simulink model "SecRwLtStBkReclnIsPosChk"  (R2024b)
settings: Solver=FixedStepDiscrete  StartTime=0.0  StopTime=10.0  FixedStep=0.01  RelTol=1e-3
undefined symbols (not defined in the file or in its folder): KeSMSuSecRwStBackPosDelta_Val, KeSMSuSecRwStBackPosTolr_Val, KeSMSuVehicleModelConfig_Val
libraries: StIsPosChkLib x13, simulink x7
(part 2 of 2)

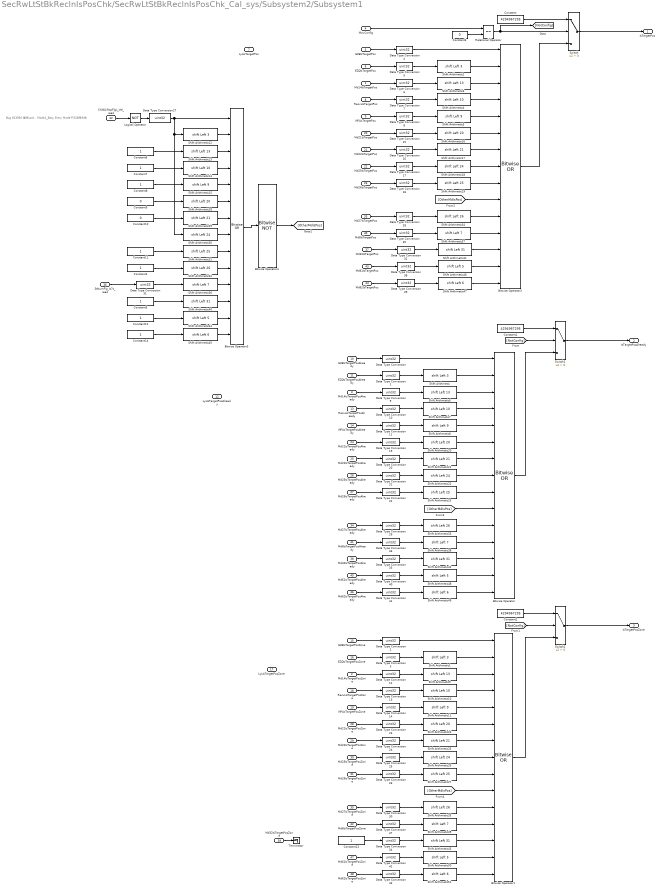
== system SecRwLtStBkReclnIsPosChk/SecRwLtStBkReclnIsPosChk_Cal_sys/Subsystem2/Subsystem1 ==
  note: Bug 813950 童锁Lock，Mode1_Easy Entry Mode 不应调用失败
  Md14IsTargetPos : Inport
  Md14IsTargetPosZone : Inport  Port=2
  Md14IsTargetPosAlready : Inport  Port=3
  MovConfig : Inport  Port=4
  EZEIsTargetPos : Inport  Port=5
  EZQIsTargetPos : Inport  Port=6
  LyLIsTargetPos : Inport  Port=7
  RecvLIsTargetPos : Inport  Port=8
  VIPLIsTargetPos : Inport  Port=9
  EZEIsTargetPosAlready : Inport  Port=10
  EZQIsTargetPosAlready : Inport  Port=11
  LyLIsTargetPosAlready : Inport  Port=12
  RecvLIsTargetPosAlready : Inport  Port=13
  VIPLIsTargetPosAlready : Inport  Port=14
  EZEIsTargetPosZone : Inport  Port=15
  EZQIsTargetPosZone : Inport  Port=16
  LyLIsTargetPosZone : Inport  Port=17
  RecvLIsTargetPosZone : Inport  Port=18
  VIPLIsTargetPosZone : Inport  Port=19
  Md21IsTargetPos : Inport  Port=20
  Md22IsTargetPos : Inport  Port=21
  Md25IsTargetPos : Inport  Port=22
  Md26IsTargetPos : Inport  Port=23
  Md21IsTargetPosAlready : Inport  Port=24
  Md22IsTargetPosAlready : Inport  Port=25
  Md25IsTargetPosAlready : Inport  Port=26
  Md26IsTargetPosAlready : Inport  Port=27
  Md21IsTargetPosZone : Inport  Port=28
  Md22IsTargetPosZone : Inport  Port=29
  Md25IsTargetPosZone : Inport  Port=30
  Md26IsTargetPosZone : Inport  Port=31
  ChldLkRspFlgL_Val_read : Inport  Port=32
  Md27IsTargetPos : Inport  Port=33
  Md27IsTargetPosAlready : Inport  Port=34
  Md27IsTargetPosZone : Inport  Port=35
  StNumFlg_Is7s_read : Inport  Port=36
  Md32IsTargetPos : Inport  Port=37
  Md32IsTargetPosAlready : Inport  Port=38
  Md32IsTargetPosZone : Inport  Port=39
  Md8IsTargetPos : Inport  Port=40
  Md8IsTargetPosAlready : Inport  Port=41
  Md8IsTargetPosZone : Inport  Port=42
  Md61IsTargetPos : Inport  Port=43
  Md62IsTargetPos : Inport  Port=44
  Md61IsTargetPosAlready : Inport  Port=45
  Md62IsTargetPosAlready : Inport  Port=46
  Md61IsTargetPosZone : Inport  Port=47
  Md62IsTargetPosZone : Inport  Port=48
  Bitwise Operator : simulink/Logic and Bit Operations/Bitwise Operator  logicop=OR  UseBitMask=off  NumInputPorts=15  BitMask=bin2dec('11011001')  BitMaskRealWorld=Stored Integer
  Bitwise Operator1 : simulink/Logic and Bit Operations/Bitwise Operator  logicop=OR  UseBitMask=off  NumInputPorts=15  BitMask=bin2dec('11011001')  BitMaskRealWorld=Stored Integer
  Bitwise Operator2 : simulink/Logic and Bit Operations/Bitwise Operator  logicop=OR  UseBitMask=off  NumInputPorts=15  BitMask=bin2dec('11011001')  BitMaskRealWorld=Stored Integer
  Bitwise Operator3 : simulink/Logic and Bit Operations/Bitwise Operator  logicop=OR  UseBitMask=off  NumInputPorts=14  BitMask=bin2dec('11011001')  BitMaskRealWorld=Stored Integer
  Bitwise Operator4 : simulink/Logic and Bit Operations/Bitwise Operator  logicop=NOT  UseBitMask=off  BitMask=bin2dec('11011001')  BitMaskRealWorld=Stored Integer
  Constant : Constant  Value=4294967295  OutDataTypeStr=uint32
  Constant1 : Constant  Value=4294967295  OutDataTypeStr=uint32
  Constant10 : Constant  Value=0  OutDataTypeStr=uint32
  Constant{4..8,11..14} (9 alike) : Constant  OutDataTypeStr=uint32
  Constant2 : Constant  Value=4294967295  OutDataTypeStr=uint32
  Constant3 : Constant  Value=0  OutDataTypeStr=uint8
  Constant9 : Constant  Value=0  OutDataTypeStr=uint32
  Data Type Conversion{,1..43} (44 alike) : DataTypeConversion  OutDataTypeStr=uint32  SaturateOnIntegerOverflow=off  RndMeth=Floor
  Logical Operator : Logic  Operator=NOT  AllPortsSameDT=off  OutDataTypeStr=boolean
  Relational Operator : RelationalOperator  Operator===  OutDataTypeStr=boolean  RndMeth=Simplest  InputSameDT=off
  Shift Arithmetic{,1..2,12} (4 alike) : ArithShift  BitShiftNumber=3  BitShiftDirection=Left
  Shift Arithmetic{4,7,10,14} (4 alike) : ArithShift  BitShiftNumber=10  BitShiftDirection=Left
  Shift Arithmetic{5,8,11,15} (4 alike) : ArithShift  BitShiftNumber=9  BitShiftDirection=Left
  Shift Arithmetic{3,6,9,13} (4 alike) : ArithShift  BitShiftNumber=13  BitShiftDirection=Left
  Shift Arithmetic{16,20,24,28} (4 alike) : ArithShift  BitShiftNumber=20  BitShiftDirection=Left
  Shift Arithmetic{17,21,25,29} (4 alike) : ArithShift  BitShiftNumber=21  BitShiftDirection=Left
  Shift Arithmetic{18,22,26,30} (4 alike) : ArithShift  BitShiftNumber=24  BitShiftDirection=Left
  Shift Arithmetic{19,23,27,31} (4 alike) : ArithShift  BitShiftNumber=25  BitShiftDirection=Left
  Shift Arithmetic{32..35} (4 alike) : ArithShift  BitShiftNumber=26  BitShiftDirection=Left
  Shift Arithmetic{36..39} (4 alike) : ArithShift  BitShiftNumber=7  BitShiftDirection=Left
  Shift Arithmetic{40..43} (4 alike) : ArithShift  BitShiftNumber=31  BitShiftDirection=Left
  Shift Arithmetic{44,46,48,50} (4 alike) : ArithShift  BitShiftNumber=5  BitShiftDirection=Left
  Shift Arithmetic{45,47,49,51} (4 alike) : ArithShift  BitShiftNumber=6  BitShiftDirection=Left
  Switch : Switch  Criteria=u2 > Threshold  SaturateOnIntegerOverflow=off  InputSameDT=off
  Switch1 : Switch  Criteria=u2 > Threshold  SaturateOnIntegerOverflow=off  InputSameDT=off
  Switch2 : Switch  Criteria=u2 > Threshold  SaturateOnIntegerOverflow=off  InputSameDT=off
  Terminator : Terminator
  IsTargetPos : Outport  VectorParamsAs1DForOutWhenUnconnected=off
      settings: EnsureOutportIsVirtual=on
  IsTargetPosAlready : Outport  Port=2  VectorParamsAs1DForOutWhenUnconnected=off
      settings: EnsureOutportIsVirtual=on
  IsTargetPosZone : Outport  Port=3  VectorParamsAs1DForOutWhenUnconnected=off
      settings: EnsureOutportIsVirtual=on
  wires:
  Constant3/1 -> Relational Operator/2
  Constant/1 -> Switch/1
  Relational Operator/1 -> [NotConfig], Switch/2
  MovConfig/1 -> Relational Operator/1
  Switch/1 -> IsTargetPos/1
  [NotConfig] -> Switch1/2
  Constant1/1 -> Switch1/1
  Switch1/1 -> IsTargetPosAlready/1
  Switch2/1 -> IsTargetPosZone/1
  Constant2/1 -> Switch2/1
  [NotConfig] -> Switch2/2
  Data Type Conversion1/1 -> Shift Arithmetic/1
  Data Type Conversion/1 -> Bitwise Operator/1
  Shift Arithmetic/1 -> Bitwise Operator/2
  Shift Arithmetic1/1 -> Bitwise Operator1/2
  Data Type Conversion2/1 -> Bitwise Operator1/1
  Data Type Conversion3/1 -> Shift Arithmetic1/1
  Bitwise Operator1/1 -> Switch2/3
  Bitwise Operator/1 -> Switch1/3
  Shift Arithmetic2/1 -> Bitwise Operator2/2
  Data Type Conversion4/1 -> Bitwise Operator2/1
  Data Type Conversion5/1 -> Shift Arithmetic2/1
  Bitwise Operator2/1 -> Switch/3
  EZEIsTargetPos/1 -> Data Type Conversion4/1
  EZQIsTargetPos/1 -> Data Type Conversion5/1
  EZQIsTargetPosZone/1 -> Data Type Conversion3/1
  EZEIsTargetPosZone/1 -> Data Type Conversion2/1
  EZQIsTargetPosAlready/1 -> Data Type Conversion1/1
  EZEIsTargetPosAlready/1 -> Data Type Conversion/1
  Shift Arithmetic3/1 -> Bitwise Operator2/3
  Shift Arithmetic4/1 -> Bitwise Operator2/4
  Shift Arithmetic5/1 -> Bitwise Operator2/5
  Data Type Conversion7/1 -> Shift Arithmetic4/1
  Data Type Conversion6/1 -> Shift Arithmetic3/1
  Data Type Conversion8/1 -> Shift Arithmetic5/1
  RecvLIsTargetPos/1 -> Data Type Conversion7/1
  VIPLIsTargetPos/1 -> Data Type Conversion8/1
  VIPLIsTargetPosAlready/1 -> Data Type Conversion11/1
  RecvLIsTargetPosAlready/1 -> Data Type Conversion10/1
  Data Type Conversion11/1 -> Shift Arithmetic8/1
  Data Type Conversion9/1 -> Shift Arithmetic6/1
  Data Type Conversion10/1 -> Shift Arithmetic7/1
  Shift Arithmetic8/1 -> Bitwise Operator/5
  Shift Arithmetic7/1 -> Bitwise Operator/4
  Shift Arithmetic6/1 -> Bitwise Operator/3
  Data Type Conversion14/1 -> Shift Arithmetic11/1
  Data Type Conversion13/1 -> Shift Arithmetic10/1
  VIPLIsTargetPosZone/1 -> Data Type Conversion14/1
  Shift Arithmetic10/1 -> Bitwise Operator1/4
  RecvLIsTargetPosZone/1 -> Data Type Conversion13/1
  Shift Arithmetic9/1 -> Bitwise Operator1/3
  Shift Arithmetic11/1 -> Bitwise Operator1/5
  Data Type Conversion12/1 -> Shift Arithmetic9/1
  Constant6/1 -> Shift Arithmetic13/1
  Constant7/1 -> Shift Arithmetic14/1
  Constant8/1 -> Shift Arithmetic15/1
  Shift Arithmetic12/1 -> Bitwise Operator3/2
  Shift Arithmetic13/1 -> Bitwise Operator3/3
  Shift Arithmetic14/1 -> Bitwise Operator3/4
  Shift Arithmetic15/1 -> Bitwise Operator3/5
  ChldLkRspFlgL_Val_read/1 -> Logical Operator/1
  Bitwise Operator3/1 -> Bitwise Operator4/1
  Bitwise Operator4/1 -> [OtherMdIsPos]
  [OtherMdIsPos] -> Bitwise Operator2/10
  Md26IsTargetPos/1 -> Data Type Conversion18/1
  Md22IsTargetPos/1 -> Data Type Conversion16/1
  Md25IsTargetPos/1 -> Data Type Conversion17/1
  Md21IsTargetPos/1 -> Data Type Conversion15/1
  Data Type Conversion15/1 -> Shift Arithmetic16/1
  Data Type Conversion16/1 -> Shift Arithmetic17/1
  Data Type Conversion17/1 -> Shift Arithmetic18/1
  Data Type Conversion18/1 -> Shift Arithmetic19/1
  Shift Arithmetic16/1 -> Bitwise Operator2/6
  Shift Arithmetic17/1 -> Bitwise Operator2/7
  Shift Arithmetic18/1 -> Bitwise Operator2/8
  Shift Arithmetic19/1 -> Bitwise Operator2/9
  [OtherMdIsPos] -> Bitwise Operator/10
  [OtherMdIsPos] -> Bitwise Operator1/10
  Data Type Conversion22/1 -> Shift Arithmetic23/1
  Data Type Conversion19/1 -> Shift Arithmetic20/1
  Md21IsTargetPosAlready/1 -> Data Type Conversion19/1
  Shift Arithmetic23/1 -> Bitwise Operator/9
  Data Type Conversion20/1 -> Shift Arithmetic21/1
  Md25IsTargetPosAlready/1 -> Data Type Conversion21/1
  Shift Arithmetic22/1 -> Bitwise Operator/8
  Data Type Conversion21/1 -> Shift Arithmetic22/1
  Shift Arithmetic21/1 -> Bitwise Operator/7
  Md22IsTargetPosAlready/1 -> Data Type Conversion20/1
  Md26IsTargetPosAlready/1 -> Data Type Conversion22/1
  Shift Arithmetic20/1 -> Bitwise Operator/6
  Data Type Conversion26/1 -> Shift Arithmetic27/1
  Data Type Conversion23/1 -> Shift Arithmetic24/1
  Md21IsTargetPosZone/1 -> Data Type Conversion23/1
  Shift Arithmetic27/1 -> Bitwise Operator1/9
  Data Type Conversion24/1 -> Shift Arithmetic25/1
  Shift Arithmetic26/1 -> Bitwise Operator1/8
  Data Type Conversion25/1 -> Shift Arithmetic26/1
  Shift Arithmetic25/1 -> Bitwise Operator1/7
  Md22IsTargetPosZone/1 -> Data Type Conversion24/1
  Md26IsTargetPosZone/1 -> Data Type Conversion26/1
  Shift Arithmetic24/1 -> Bitwise Operator1/6
  Constant9/1 -> Shift Arithmetic28/1
  Shift Arithmetic28/1 -> Bitwise Operator3/6
  Shift Arithmetic29/1 -> Bitwise Operator3/7
  Constant10/1 -> Shift Arithmetic29/1
  Constant11/1 -> Shift Arithmetic31/1
  Shift Arithmetic30/1 -> Bitwise Operator3/8
  Shift Arithmetic31/1 -> Bitwise Operator3/9
  Data Type Conversion27/1 -> Shift Arithmetic30/1, Shift Arithmetic12/1, Bitwise Operator3/1
  Logical Operator/1 -> Data Type Conversion27/1
  Shift Arithmetic32/1 -> Bitwise Operator3/10
  Constant4/1 -> Shift Arithmetic32/1
  Shift Arithmetic34/1 -> Bitwise Operator2/11
  Data Type Conversion28/1 -> Shift Arithmetic34/1
  Md27IsTargetPos/1 -> Data Type Conversion28/1
  Md27IsTargetPosAlready/1 -> Data Type Conversion29/1
  Data Type Conversion29/1 -> Shift Arithmetic33/1
  Shift Arithmetic33/1 -> Bitwise Operator/11
  Shift Arithmetic35/1 -> Bitwise Operator1/11
  Data Type Conversion30/1 -> Shift Arithmetic35/1
  Md27IsTargetPosZone/1 -> Data Type Conversion30/1
  Shift Arithmetic36/1 -> Bitwise Operator3/11
  StNumFlg_Is7s_read/1 -> Data Type Conversion31/1
  Shift Arithmetic37/1 -> Bitwise Operator2/12
  Shift Arithmetic38/1 -> Bitwise Operator/12
  Shift Arithmetic39/1 -> Bitwise Operator1/12
  Data Type Conversion31/1 -> Shift Arithmetic36/1
  Constant5/1 -> Shift Arithmetic40/1
  Shift Arithmetic40/1 -> Bitwise Operator3/12
  Shift Arithmetic41/1 -> Bitwise Operator2/13
  Data Type Conversion32/1 -> Shift Arithmetic41/1
  Md32IsTargetPos/1 -> Data Type Conversion32/1
  Shift Arithmetic42/1 -> Bitwise Operator/13
  Md32IsTargetPosAlready/1 -> Data Type Conversion33/1
  Data Type Conversion33/1 -> Shift Arithmetic42/1
  Data Type Conversion34/1 -> Shift Arithmetic43/1
  Shift Arithmetic43/1 -> Bitwise Operator1/13
  Md8IsTargetPos/1 -> Data Type Conversion35/1
  Data Type Conversion35/1 -> Shift Arithmetic37/1
  Data Type Conversion36/1 -> Shift Arithmetic38/1
  Md8IsTargetPosAlready/1 -> Data Type Conversion36/1
  Md8IsTargetPosZone/1 -> Data Type Conversion37/1
  Data Type Conversion37/1 -> Shift Arithmetic39/1
  Md32IsTargetPosZone/1 -> Terminator/1
  Constant13/1 -> Data Type Conversion34/1
  Md25IsTargetPosZone/1 -> Data Type Conversion25/1
  Shift Arithmetic45/1 -> Bitwise Operator3/14
  Shift Arithmetic44/1 -> Bitwise Operator3/13
  Constant12/1 -> Shift Arithmetic44/1
  Constant14/1 -> Shift Arithmetic45/1
  Md61IsTargetPos/1 -> Data Type Conversion38/1
  Data Type Conversion38/1 -> Shift Arithmetic46/1
  Shift Arithmetic46/1 -> Bitwise Operator2/14
  Shift Arithmetic47/1 -> Bitwise Operator2/15
  Data Type Conversion39/1 -> Shift Arithmetic47/1
  Md62IsTargetPos/1 -> Data Type Conversion39/1
  Data Type Conversion40/1 -> Shift Arithmetic48/1
  Md61IsTargetPosAlready/1 -> Data Type Conversion40/1
  Shift Arithmetic48/1 -> Bitwise Operator/14
  Shift Arithmetic49/1 -> Bitwise Operator/15
  Md62IsTargetPosAlready/1 -> Data Type Conversion41/1
  Data Type Conversion41/1 -> Shift Arithmetic49/1
  Md61IsTargetPosZone/1 -> Data Type Conversion42/1
  Shift Arithmetic50/1 -> Bitwise Operator1/14
  Data Type Conversion42/1 -> Shift Arithmetic50/1
  Data Type Conversion43/1 -> Shift Arithmetic51/1
  Shift Arithmetic51/1 -> Bitwise Operator1/15
  Md62IsTargetPosZone/1 -> Data Type Conversion43/1
  Md14IsTargetPos/1 -> Data Type Conversion6/1
  Md14IsTargetPosAlready/1 -> Data Type Conversion9/1
  Md14IsTargetPosZone/1 -> Data Type Conversion12/1

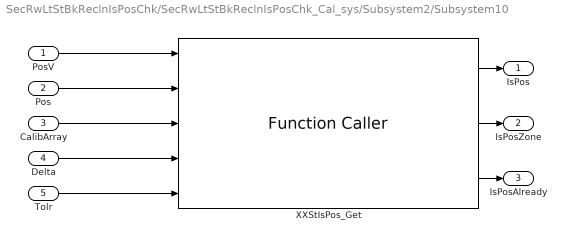
== system SecRwLtStBkReclnIsPosChk/SecRwLtStBkReclnIsPosChk_Cal_sys/Subsystem2/Subsystem10 ==
  PosV : Inport
  Pos : Inport  Port=2
  CalibArray : Inport  Port=3
  Delta : Inport  Port=4
  Tolr : Inport  Port=5
  XXStIsPos_Get : FunctionCaller  FunctionPrototype=[IsPos,IsPosZone,IsPosAlready] = XXStIsPos_Get(PosV,Pos,CalibArray,Delta,Tolr)  InputArgumentSpecifications=boolean(true), uint16(1), uint16([1;1;1]), uint16(1), uint16(1)  OutputArgumentSpecifications=boolean(true), boolean(true), boolean(true)
  IsPos : Outport  VectorParamsAs1DForOutWhenUnconnected=off
  IsPosZone : Outport  Port=2  VectorParamsAs1DForOutWhenUnconnected=off
  IsPosAlready : Outport  Port=3  VectorParamsAs1DForOutWhenUnconnected=off
  wires:
  XXStIsPos_Get/3 -> IsPosAlready/1
  CalibArray/1 -> XXStIsPos_Get/3
  XXStIsPos_Get/1 -> IsPos/1
  Pos/1 -> XXStIsPos_Get/2
  XXStIsPos_Get/2 -> IsPosZone/1
  PosV/1 -> XXStIsPos_Get/1
  Tolr/1 -> XXStIsPos_Get/5
  Delta/1 -> XXStIsPos_Get/4

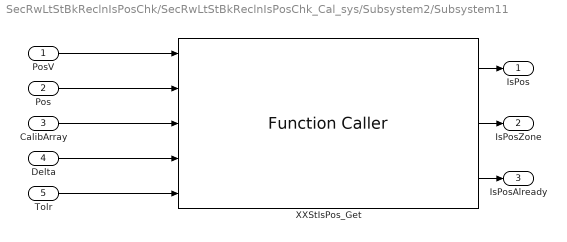
== system SecRwLtStBkReclnIsPosChk/SecRwLtStBkReclnIsPosChk_Cal_sys/Subsystem2/Subsystem11 ==
  PosV : Inport
  Pos : Inport  Port=2
  CalibArray : Inport  Port=3
  Delta : Inport  Port=4
  Tolr : Inport  Port=5
  XXStIsPos_Get : FunctionCaller  FunctionPrototype=[IsPos,IsPosZone,IsPosAlready] = XXStIsPos_Get(PosV,Pos,CalibArray,Delta,Tolr)  InputArgumentSpecifications=boolean(true), uint16(1), uint16([1;1;1]), uint16(1), uint16(1)  OutputArgumentSpecifications=boolean(true), boolean(true), boolean(true)
  IsPos : Outport  VectorParamsAs1DForOutWhenUnconnected=off
  IsPosZone : Outport  Port=2  VectorParamsAs1DForOutWhenUnconnected=off
  IsPosAlready : Outport  Port=3  VectorParamsAs1DForOutWhenUnconnected=off
  wires:
  Delta/1 -> XXStIsPos_Get/4
  Tolr/1 -> XXStIsPos_Get/5
  PosV/1 -> XXStIsPos_Get/1
  XXStIsPos_Get/2 -> IsPosZone/1
  Pos/1 -> XXStIsPos_Get/2
  XXStIsPos_Get/1 -> IsPos/1
  CalibArray/1 -> XXStIsPos_Get/3
  XXStIsPos_Get/3 -> IsPosAlready/1

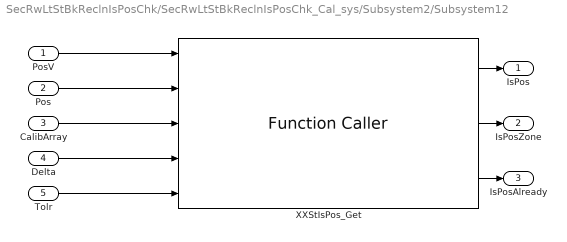
== system SecRwLtStBkReclnIsPosChk/SecRwLtStBkReclnIsPosChk_Cal_sys/Subsystem2/Subsystem12 ==
  PosV : Inport
  Pos : Inport  Port=2
  CalibArray : Inport  Port=3
  Delta : Inport  Port=4
  Tolr : Inport  Port=5
  XXStIsPos_Get : FunctionCaller  FunctionPrototype=[IsPos,IsPosZone,IsPosAlready] = XXStIsPos_Get(PosV,Pos,CalibArray,Delta,Tolr)  InputArgumentSpecifications=boolean(true), uint16(1), uint16([1;1;1]), uint16(1), uint16(1)  OutputArgumentSpecifications=boolean(true), boolean(true), boolean(true)
  IsPos : Outport  VectorParamsAs1DForOutWhenUnconnected=off
  IsPosZone : Outport  Port=2  VectorParamsAs1DForOutWhenUnconnected=off
  IsPosAlready : Outport  Port=3  VectorParamsAs1DForOutWhenUnconnected=off
  wires:
  XXStIsPos_Get/3 -> IsPosAlready/1
  CalibArray/1 -> XXStIsPos_Get/3
  XXStIsPos_Get/1 -> IsPos/1
  Pos/1 -> XXStIsPos_Get/2
  XXStIsPos_Get/2 -> IsPosZone/1
  PosV/1 -> XXStIsPos_Get/1
  Tolr/1 -> XXStIsPos_Get/5
  Delta/1 -> XXStIsPos_Get/4

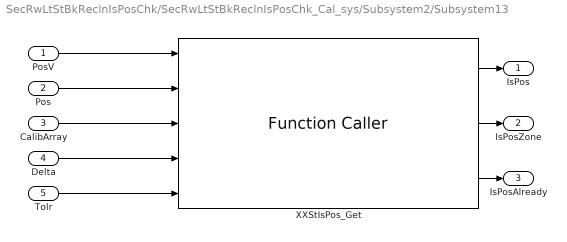
== system SecRwLtStBkReclnIsPosChk/SecRwLtStBkReclnIsPosChk_Cal_sys/Subsystem2/Subsystem13 ==
  PosV : Inport
  Pos : Inport  Port=2
  CalibArray : Inport  Port=3
  Delta : Inport  Port=4
  Tolr : Inport  Port=5
  XXStIsPos_Get : FunctionCaller  FunctionPrototype=[IsPos,IsPosZone,IsPosAlready] = XXStIsPos_Get(PosV,Pos,CalibArray,Delta,Tolr)  InputArgumentSpecifications=boolean(true), uint16(1), uint16([1;1;1]), uint16(1), uint16(1)  OutputArgumentSpecifications=boolean(true), boolean(true), boolean(true)
  IsPos : Outport  VectorParamsAs1DForOutWhenUnconnected=off
  IsPosZone : Outport  Port=2  VectorParamsAs1DForOutWhenUnconnected=off
  IsPosAlready : Outport  Port=3  VectorParamsAs1DForOutWhenUnconnected=off
  wires:
  Delta/1 -> XXStIsPos_Get/4
  Tolr/1 -> XXStIsPos_Get/5
  PosV/1 -> XXStIsPos_Get/1
  XXStIsPos_Get/2 -> IsPosZone/1
  Pos/1 -> XXStIsPos_Get/2
  XXStIsPos_Get/1 -> IsPos/1
  CalibArray/1 -> XXStIsPos_Get/3
  XXStIsPos_Get/3 -> IsPosAlready/1

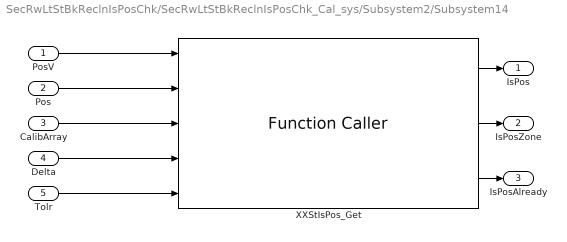
== system SecRwLtStBkReclnIsPosChk/SecRwLtStBkReclnIsPosChk_Cal_sys/Subsystem2/Subsystem14 ==
  PosV : Inport
  Pos : Inport  Port=2
  CalibArray : Inport  Port=3
  Delta : Inport  Port=4
  Tolr : Inport  Port=5
  XXStIsPos_Get : FunctionCaller  FunctionPrototype=[IsPos,IsPosZone,IsPosAlready] = XXStIsPos_Get(PosV,Pos,CalibArray,Delta,Tolr)  InputArgumentSpecifications=boolean(true), uint16(1), uint16([1;1;1]), uint16(1), uint16(1)  OutputArgumentSpecifications=boolean(true), boolean(true), boolean(true)
  IsPos : Outport  VectorParamsAs1DForOutWhenUnconnected=off
  IsPosZone : Outport  Port=2  VectorParamsAs1DForOutWhenUnconnected=off
  IsPosAlready : Outport  Port=3  VectorParamsAs1DForOutWhenUnconnected=off
  wires:
  XXStIsPos_Get/3 -> IsPosAlready/1
  CalibArray/1 -> XXStIsPos_Get/3
  XXStIsPos_Get/1 -> IsPos/1
  Pos/1 -> XXStIsPos_Get/2
  XXStIsPos_Get/2 -> IsPosZone/1
  PosV/1 -> XXStIsPos_Get/1
  Tolr/1 -> XXStIsPos_Get/5
  Delta/1 -> XXStIsPos_Get/4

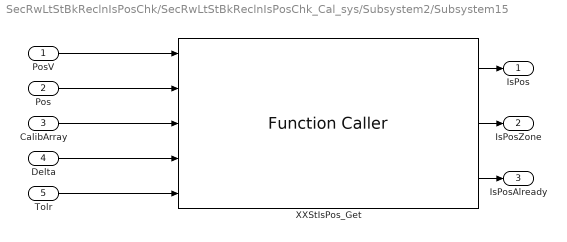
== system SecRwLtStBkReclnIsPosChk/SecRwLtStBkReclnIsPosChk_Cal_sys/Subsystem2/Subsystem15 ==
  PosV : Inport
  Pos : Inport  Port=2
  CalibArray : Inport  Port=3
  Delta : Inport  Port=4
  Tolr : Inport  Port=5
  XXStIsPos_Get : FunctionCaller  FunctionPrototype=[IsPos,IsPosZone,IsPosAlready] = XXStIsPos_Get(PosV,Pos,CalibArray,Delta,Tolr)  InputArgumentSpecifications=boolean(true), uint16(1), uint16([1;1;1]), uint16(1), uint16(1)  OutputArgumentSpecifications=boolean(true), boolean(true), boolean(true)
  IsPos : Outport  VectorParamsAs1DForOutWhenUnconnected=off
  IsPosZone : Outport  Port=2  VectorParamsAs1DForOutWhenUnconnected=off
  IsPosAlready : Outport  Port=3  VectorParamsAs1DForOutWhenUnconnected=off
  wires:
  Delta/1 -> XXStIsPos_Get/4
  Tolr/1 -> XXStIsPos_Get/5
  PosV/1 -> XXStIsPos_Get/1
  XXStIsPos_Get/2 -> IsPosZone/1
  Pos/1 -> XXStIsPos_Get/2
  XXStIsPos_Get/1 -> IsPos/1
  CalibArray/1 -> XXStIsPos_Get/3
  XXStIsPos_Get/3 -> IsPosAlready/1

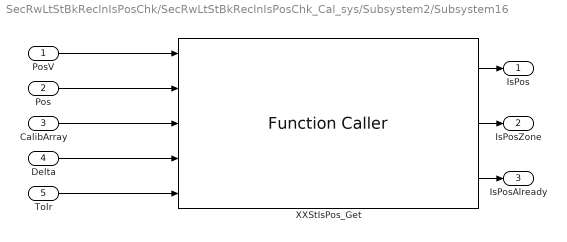
== system SecRwLtStBkReclnIsPosChk/SecRwLtStBkReclnIsPosChk_Cal_sys/Subsystem2/Subsystem16 ==
  PosV : Inport
  Pos : Inport  Port=2
  CalibArray : Inport  Port=3
  Delta : Inport  Port=4
  Tolr : Inport  Port=5
  XXStIsPos_Get : FunctionCaller  FunctionPrototype=[IsPos,IsPosZone,IsPosAlready] = XXStIsPos_Get(PosV,Pos,CalibArray,Delta,Tolr)  InputArgumentSpecifications=boolean(true), uint16(1), uint16([1;1;1]), uint16(1), uint16(1)  OutputArgumentSpecifications=boolean(true), boolean(true), boolean(true)
  IsPos : Outport  VectorParamsAs1DForOutWhenUnconnected=off
  IsPosZone : Outport  Port=2  VectorParamsAs1DForOutWhenUnconnected=off
  IsPosAlready : Outport  Port=3  VectorParamsAs1DForOutWhenUnconnected=off
  wires:
  XXStIsPos_Get/3 -> IsPosAlready/1
  CalibArray/1 -> XXStIsPos_Get/3
  XXStIsPos_Get/1 -> IsPos/1
  Pos/1 -> XXStIsPos_Get/2
  XXStIsPos_Get/2 -> IsPosZone/1
  PosV/1 -> XXStIsPos_Get/1
  Tolr/1 -> XXStIsPos_Get/5
  Delta/1 -> XXStIsPos_Get/4

== system SecRwLtStBkReclnIsPosChk/SecRwLtStBkReclnIsPosChk_Cal_sys/Subsystem2/Subsystem17 ==
  PosV : Inport
  Pos : Inport  Port=2
  CalibArray : Inport  Port=3
  Delta : Inport  Port=4
  Tolr : Inport  Port=5
  XXStIsPos_Get : FunctionCaller  FunctionPrototype=[IsPos,IsPosZone,IsPosAlready] = XXStIsPos_Get(PosV,Pos,CalibArray,Delta,Tolr)  InputArgumentSpecifications=boolean(true), uint16(1), uint16([1;1;1]), uint16(1), uint16(1)  OutputArgumentSpecifications=boolean(true), boolean(true), boolean(true)
  IsPos : Outport  VectorParamsAs1DForOutWhenUnconnected=off
  IsPosZone : Outport  Port=2  VectorParamsAs1DForOutWhenUnconnected=off
  IsPosAlready : Outport  Port=3  VectorParamsAs1DForOutWhenUnconnected=off
  wires:
  XXStIsPos_Get/3 -> IsPosAlready/1
  CalibArray/1 -> XXStIsPos_Get/3
  XXStIsPos_Get/1 -> IsPos/1
  Pos/1 -> XXStIsPos_Get/2
  XXStIsPos_Get/2 -> IsPosZone/1
  PosV/1 -> XXStIsPos_Get/1
  Tolr/1 -> XXStIsPos_Get/5
  Delta/1 -> XXStIsPos_Get/4

== system SecRwLtStBkReclnIsPosChk/SecRwLtStBkReclnIsPosChk_Cal_sys/Subsystem2/Subsystem2 ==
  PosV : Inport
  Pos : Inport  Port=2
  CalibArray : Inport  Port=3
  Delta : Inport  Port=4
  Tolr : Inport  Port=5
  XXStIsPos_Get : FunctionCaller  FunctionPrototype=[IsPos,IsPosZone,IsPosAlready] = XXStIsPos_Get(PosV,Pos,CalibArray,Delta,Tolr)  InputArgumentSpecifications=boolean(true), uint16(1), uint16([1;1;1]), uint16(1), uint16(1)  OutputArgumentSpecifications=boolean(true), boolean(true), boolean(true)
  IsPos : Outport  VectorParamsAs1DForOutWhenUnconnected=off
  IsPosZone : Outport  Port=2  VectorParamsAs1DForOutWhenUnconnected=off
  IsPosAlready : Outport  Port=3  VectorParamsAs1DForOutWhenUnconnected=off
  wires:
  XXStIsPos_Get/3 -> IsPosAlready/1
  CalibArray/1 -> XXStIsPos_Get/3
  XXStIsPos_Get/1 -> IsPos/1
  Pos/1 -> XXStIsPos_Get/2
  XXStIsPos_Get/2 -> IsPosZone/1
  PosV/1 -> XXStIsPos_Get/1
  Tolr/1 -> XXStIsPos_Get/5
  Delta/1 -> XXStIsPos_Get/4

== system SecRwLtStBkReclnIsPosChk/SecRwLtStBkReclnIsPosChk_Cal_sys/Subsystem2/Subsystem3 ==
  PosV : Inport
  Pos : Inport  Port=2
  CalibArray : Inport  Port=3
  Delta : Inport  Port=4
  Tolr : Inport  Port=5
  XXStIsPos_Get : FunctionCaller  FunctionPrototype=[IsPos,IsPosZone,IsPosAlready] = XXStIsPos_Get(PosV,Pos,CalibArray,Delta,Tolr)  InputArgumentSpecifications=boolean(true), uint16(1), uint16([1;1;1]), uint16(1), uint16(1)  OutputArgumentSpecifications=boolean(true), boolean(true), boolean(true)
  IsPos : Outport  VectorParamsAs1DForOutWhenUnconnected=off
  IsPosZone : Outport  Port=2  VectorParamsAs1DForOutWhenUnconnected=off
  IsPosAlready : Outport  Port=3  VectorParamsAs1DForOutWhenUnconnected=off
  wires:
  Delta/1 -> XXStIsPos_Get/4
  Tolr/1 -> XXStIsPos_Get/5
  PosV/1 -> XXStIsPos_Get/1
  XXStIsPos_Get/2 -> IsPosZone/1
  Pos/1 -> XXStIsPos_Get/2
  XXStIsPos_Get/1 -> IsPos/1
  CalibArray/1 -> XXStIsPos_Get/3
  XXStIsPos_Get/3 -> IsPosAlready/1

== system SecRwLtStBkReclnIsPosChk/SecRwLtStBkReclnIsPosChk_Cal_sys/Subsystem2/Subsystem4 ==
  PosV : Inport
  Pos : Inport  Port=2
  CalibArray : Inport  Port=3
  Delta : Inport  Port=4
  Tolr : Inport  Port=5
  XXStIsPos_Get : FunctionCaller  FunctionPrototype=[IsPos,IsPosZone,IsPosAlready] = XXStIsPos_Get(PosV,Pos,CalibArray,Delta,Tolr)  InputArgumentSpecifications=boolean(true), uint16(1), uint16([1;1;1]), uint16(1), uint16(1)  OutputArgumentSpecifications=boolean(true), boolean(true), boolean(true)
  IsPos : Outport  VectorParamsAs1DForOutWhenUnconnected=off
  IsPosZone : Outport  Port=2  VectorParamsAs1DForOutWhenUnconnected=off
  IsPosAlready : Outport  Port=3  VectorParamsAs1DForOutWhenUnconnected=off
  wires:
  XXStIsPos_Get/3 -> IsPosAlready/1
  CalibArray/1 -> XXStIsPos_Get/3
  XXStIsPos_Get/1 -> IsPos/1
  Pos/1 -> XXStIsPos_Get/2
  XXStIsPos_Get/2 -> IsPosZone/1
  PosV/1 -> XXStIsPos_Get/1
  Tolr/1 -> XXStIsPos_Get/5
  Delta/1 -> XXStIsPos_Get/4

== system SecRwLtStBkReclnIsPosChk/SecRwLtStBkReclnIsPosChk_Cal_sys/Subsystem2/Subsystem5 ==
  PosV : Inport
  Pos : Inport  Port=2
  CalibArray : Inport  Port=3
  Delta : Inport  Port=4
  Tolr : Inport  Port=5
  XXStIsPos_Get : FunctionCaller  FunctionPrototype=[IsPos,IsPosZone,IsPosAlready] = XXStIsPos_Get(PosV,Pos,CalibArray,Delta,Tolr)  InputArgumentSpecifications=boolean(true), uint16(1), uint16([1;1;1]), uint16(1), uint16(1)  OutputArgumentSpecifications=boolean(true), boolean(true), boolean(true)
  IsPos : Outport  VectorParamsAs1DForOutWhenUnconnected=off
  IsPosZone : Outport  Port=2  VectorParamsAs1DForOutWhenUnconnected=off
  IsPosAlready : Outport  Port=3  VectorParamsAs1DForOutWhenUnconnected=off
  wires:
  Delta/1 -> XXStIsPos_Get/4
  Tolr/1 -> XXStIsPos_Get/5
  PosV/1 -> XXStIsPos_Get/1
  XXStIsPos_Get/2 -> IsPosZone/1
  Pos/1 -> XXStIsPos_Get/2
  XXStIsPos_Get/1 -> IsPos/1
  CalibArray/1 -> XXStIsPos_Get/3
  XXStIsPos_Get/3 -> IsPosAlready/1

== system SecRwLtStBkReclnIsPosChk/SecRwLtStBkReclnIsPosChk_Cal_sys/Subsystem2/Subsystem6 ==
  PosV : Inport
  Pos : Inport  Port=2
  CalibArray : Inport  Port=3
  Delta : Inport  Port=4
  Tolr : Inport  Port=5
  XXStIsPos_Get : FunctionCaller  FunctionPrototype=[IsPos,IsPosZone,IsPosAlready] = XXStIsPos_Get(PosV,Pos,CalibArray,Delta,Tolr)  InputArgumentSpecifications=boolean(true), uint16(1), uint16([1;1;1]), uint16(1), uint16(1)  OutputArgumentSpecifications=boolean(true), boolean(true), boolean(true)
  IsPos : Outport  VectorParamsAs1DForOutWhenUnconnected=off
  IsPosZone : Outport  Port=2  VectorParamsAs1DForOutWhenUnconnected=off
  IsPosAlready : Outport  Port=3  VectorParamsAs1DForOutWhenUnconnected=off
  wires:
  XXStIsPos_Get/3 -> IsPosAlready/1
  CalibArray/1 -> XXStIsPos_Get/3
  XXStIsPos_Get/1 -> IsPos/1
  Pos/1 -> XXStIsPos_Get/2
  XXStIsPos_Get/2 -> IsPosZone/1
  PosV/1 -> XXStIsPos_Get/1
  Tolr/1 -> XXStIsPos_Get/5
  Delta/1 -> XXStIsPos_Get/4

== system SecRwLtStBkReclnIsPosChk/SecRwLtStBkReclnIsPosChk_Cal_sys/Subsystem2/Subsystem7 ==
  PosV : Inport
  Pos : Inport  Port=2
  CalibArray : Inport  Port=3
  Delta : Inport  Port=4
  Tolr : Inport  Port=5
  XXStIsPos_Get : FunctionCaller  FunctionPrototype=[IsPos,IsPosZone,IsPosAlready] = XXStIsPos_Get(PosV,Pos,CalibArray,Delta,Tolr)  InputArgumentSpecifications=boolean(true), uint16(1), uint16([1;1;1]), uint16(1), uint16(1)  OutputArgumentSpecifications=boolean(true), boolean(true), boolean(true)
  IsPos : Outport  VectorParamsAs1DForOutWhenUnconnected=off
  IsPosZone : Outport  Port=2  VectorParamsAs1DForOutWhenUnconnected=off
  IsPosAlready : Outport  Port=3  VectorParamsAs1DForOutWhenUnconnected=off
  wires:
  Delta/1 -> XXStIsPos_Get/4
  Tolr/1 -> XXStIsPos_Get/5
  PosV/1 -> XXStIsPos_Get/1
  XXStIsPos_Get/2 -> IsPosZone/1
  Pos/1 -> XXStIsPos_Get/2
  XXStIsPos_Get/1 -> IsPos/1
  CalibArray/1 -> XXStIsPos_Get/3
  XXStIsPos_Get/3 -> IsPosAlready/1

== system SecRwLtStBkReclnIsPosChk/SecRwLtStBkReclnIsPosChk_Cal_sys/Subsystem2/Subsystem8 ==
  PosV : Inport
  Pos : Inport  Port=2
  CalibArray : Inport  Port=3
  Delta : Inport  Port=4
  Tolr : Inport  Port=5
  XXStIsPos_Get : FunctionCaller  FunctionPrototype=[IsPos,IsPosZone,IsPosAlready] = XXStIsPos_Get(PosV,Pos,CalibArray,Delta,Tolr)  InputArgumentSpecifications=boolean(true), uint16(1), uint16([1;1;1]), uint16(1), uint16(1)  OutputArgumentSpecifications=boolean(true), boolean(true), boolean(true)
  IsPos : Outport  VectorParamsAs1DForOutWhenUnconnected=off
  IsPosZone : Outport  Port=2  VectorParamsAs1DForOutWhenUnconnected=off
  IsPosAlready : Outport  Port=3  VectorParamsAs1DForOutWhenUnconnected=off
  wires:
  XXStIsPos_Get/3 -> IsPosAlready/1
  CalibArray/1 -> XXStIsPos_Get/3
  XXStIsPos_Get/1 -> IsPos/1
  Pos/1 -> XXStIsPos_Get/2
  XXStIsPos_Get/2 -> IsPosZone/1
  PosV/1 -> XXStIsPos_Get/1
  Tolr/1 -> XXStIsPos_Get/5
  Delta/1 -> XXStIsPos_Get/4

== system SecRwLtStBkReclnIsPosChk/SecRwLtStBkReclnIsPosChk_Cal_sys/Subsystem2/Subsystem9 ==
  PosV : Inport
  Pos : Inport  Port=2
  CalibArray : Inport  Port=3
  Delta : Inport  Port=4
  Tolr : Inport  Port=5
  XXStIsPos_Get : FunctionCaller  FunctionPrototype=[IsPos,IsPosZone,IsPosAlready] = XXStIsPos_Get(PosV,Pos,CalibArray,Delta,Tolr)  InputArgumentSpecifications=boolean(true), uint16(1), uint16([1;1;1]), uint16(1), uint16(1)  OutputArgumentSpecifications=boolean(true), boolean(true), boolean(true)
  IsPos : Outport  VectorParamsAs1DForOutWhenUnconnected=off
  IsPosZone : Outport  Port=2  VectorParamsAs1DForOutWhenUnconnected=off
  IsPosAlready : Outport  Port=3  VectorParamsAs1DForOutWhenUnconnected=off
  wires:
  Delta/1 -> XXStIsPos_Get/4
  Tolr/1 -> XXStIsPos_Get/5
  PosV/1 -> XXStIsPos_Get/1
  XXStIsPos_Get/2 -> IsPosZone/1
  Pos/1 -> XXStIsPos_Get/2
  XXStIsPos_Get/1 -> IsPos/1
  CalibArray/1 -> XXStIsPos_Get/3
  XXStIsPos_Get/3 -> IsPosAlready/1
